simulink model "test1"  (R2015a)
settings: Solver=ode3  StartTime=0.0  StopTime=10.0  FixedStep=0.0001  RelTol=1e-3
settings Model: Creator=adelgayed60  LastModifiedBy=adelgayed60
settings OptimizationCC: InlineParams=on

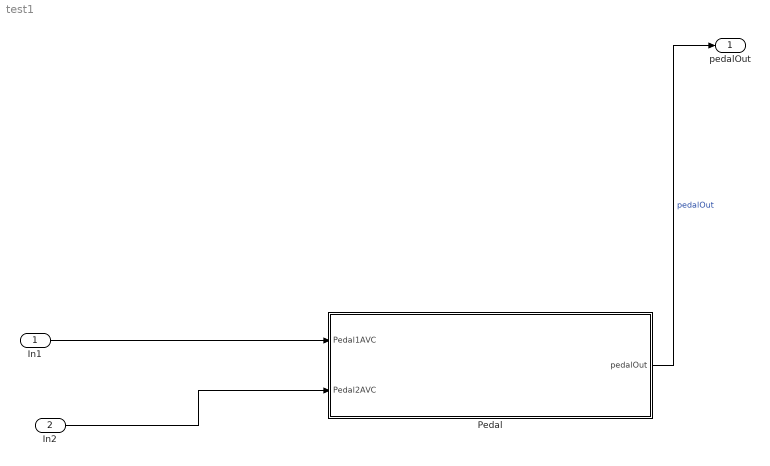
== system test1 ==
  In1 : Inport
  In2 : Inport  Port=2
  Pedal : Subsystem
  pedalOut : Outport
  wires:
  Pedal/1(pedalOut) -> pedalOut/1  "pedalOut"
  In1/1 -> Pedal/1(Pedal1AVC)
  In2/1 -> Pedal/2(Pedal2AVC)

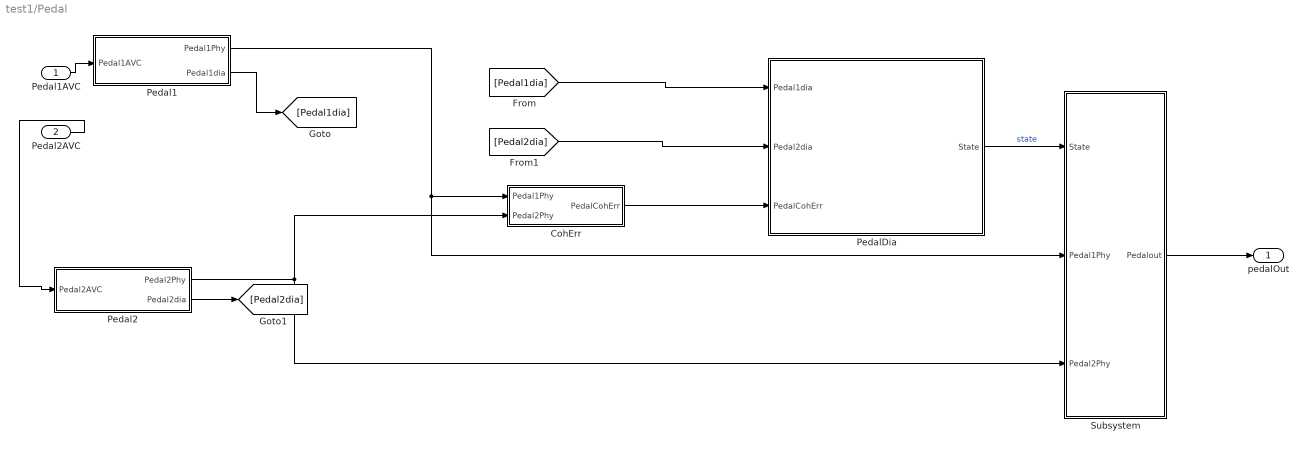
== system test1/Pedal ==
  Pedal1AVC : Inport
  Pedal2AVC : Inport  Port=2
  CohErr : Subsystem
  Pedal1 : Subsystem
  Pedal2 : Subsystem
  PedalDia : Subsystem
  Subsystem : Subsystem
  pedalOut : Outport
  wires:
  Pedal2/1(Pedal2Phy) -> CohErr/2(Pedal2Phy), Subsystem/3(Pedal2Phy)
  Subsystem/1(Pedalout) -> pedalOut/1
  Pedal2AVC/1 -> Pedal2/1(Pedal2AVC)
  Pedal2/2(Pedal2dia) -> [Pedal2dia]
  CohErr/1(PedalCohErr) -> PedalDia/3(PedalCohErr)
  [Pedal2dia] -> PedalDia/2(Pedal2dia)
  [Pedal1dia] -> PedalDia/1(Pedal1dia)
  PedalDia/1(State) -> Subsystem/1(State)  "state"
  Pedal1AVC/1 -> Pedal1/1(Pedal1AVC)
  Pedal1/2(Pedal1dia) -> [Pedal1dia]
  Pedal1/1(Pedal1Phy) -> Subsystem/2(Pedal1Phy), CohErr/1(Pedal1Phy)

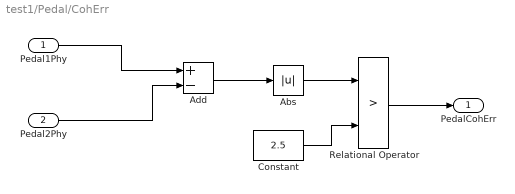
== system test1/Pedal/CohErr ==
  Pedal1Phy : Inport
  Pedal2Phy : Inport  Port=2
  Abs : Abs
  Add : Sum  Inputs=+-
  Constant : Constant  Value=2.5  OutDataTypeStr=single
  Relational Operator : RelationalOperator  Operator=>  OutDataTypeStr=boolean
  PedalCohErr : Outport
  wires:
  Pedal1Phy/1 -> Add/1
  Pedal2Phy/1 -> Add/2
  Add/1 -> Abs/1
  Abs/1 -> Relational Operator/1
  Relational Operator/1 -> PedalCohErr/1
  Constant/1 -> Relational Operator/2

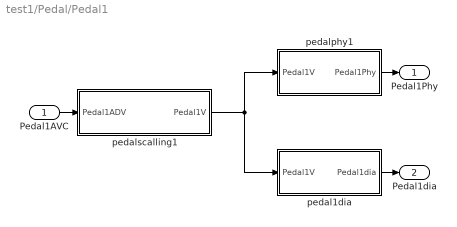
== system test1/Pedal/Pedal1 ==
  Pedal1AVC : Inport
  pedal1dia : Subsystem
  pedalphy1 : Subsystem
  pedalscalling1 : Subsystem
  Pedal1Phy : Outport
  Pedal1dia : Outport  Port=2
  wires:
  pedalscalling1/1(Pedal1V) -> pedal1dia/1(Pedal1V), pedalphy1/1(Pedal1V)
  pedal1dia/1(Pedal1dia) -> Pedal1dia/1
  pedalphy1/1(Pedal1Phy) -> Pedal1Phy/1
  Pedal1AVC/1 -> pedalscalling1/1(Pedal1ADV)

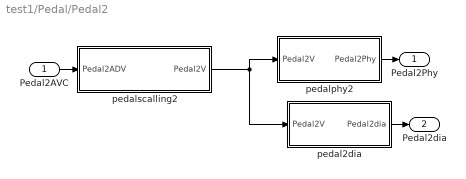
== system test1/Pedal/Pedal2 ==
  Pedal2AVC : Inport
  pedal2dia : Subsystem
  pedalphy2 : Subsystem
  pedalscalling2 : Subsystem
  Pedal2Phy : Outport
  Pedal2dia : Outport  Port=2
  wires:
  pedalscalling2/1(Pedal2V) -> pedal2dia/1(Pedal2V), pedalphy2/1(Pedal2V)
  pedalphy2/1(Pedal2Phy) -> Pedal2Phy/1
  pedal2dia/1(Pedal2dia) -> Pedal2dia/1
  Pedal2AVC/1 -> pedalscalling2/1(Pedal2ADV)

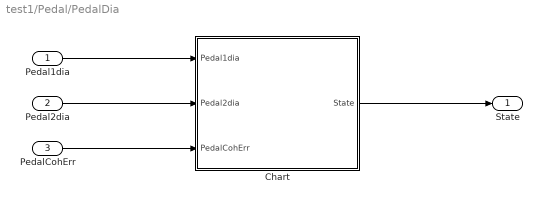
== system test1/Pedal/PedalDia ==
  Pedal1dia : Inport
  Pedal2dia : Inport  Port=2
  PedalCohErr : Inport  Port=3
  Chart : Stateflow chart  TreatAsAtomicUnit=on
  State : Outport
  wires:
  Pedal2dia/1 -> Chart/2(Pedal2dia)
  Pedal1dia/1 -> Chart/1(Pedal1dia)
  Chart/1(State) -> State/1
  PedalCohErr/1 -> Chart/3(PedalCohErr)

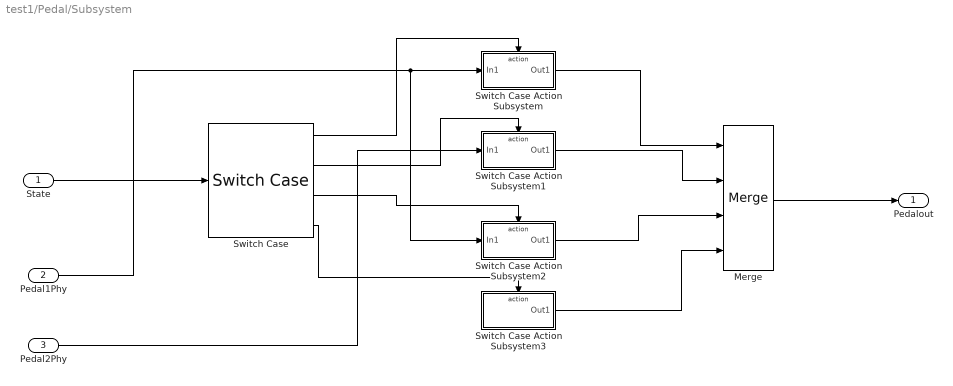
== system test1/Pedal/Subsystem ==
  State : Inport
  Pedal1Phy : Inport  Port=2
  Pedal2Phy : Inport  Port=3
  Merge : Merge  Inputs=4
  Switch Case : SwitchCase  CaseConditions={0,1,2,3}  ShowDefaultCase=off
  Switch Case Action Subsystem : Subsystem  TreatAsAtomicUnit=on
  Switch Case Action Subsystem1 : Subsystem  TreatAsAtomicUnit=on
  Switch Case Action Subsystem2 : Subsystem  TreatAsAtomicUnit=on
  Switch Case Action Subsystem3 : Subsystem  TreatAsAtomicUnit=on
  Pedalout : Outport
  wires:
  State/1 -> Switch Case/1
  Switch Case Action Subsystem/1(Out1) -> Merge/1
  Switch Case Action Subsystem1/1(Out1) -> Merge/2
  Switch Case Action Subsystem2/1(Out1) -> Merge/3
  Switch Case Action Subsystem3/1(Out1) -> Merge/4
  Switch Case/1 -> Switch Case Action Subsystem/Action
  Switch Case/2 -> Switch Case Action Subsystem1/Action
  Switch Case/3 -> Switch Case Action Subsystem2/Action
  Switch Case/4 -> Switch Case Action Subsystem3/Action
  Pedal1Phy/1 -> Switch Case Action Subsystem2/1(In1), Switch Case Action Subsystem/1(In1)
  Merge/1 -> Pedalout/1
  Pedal2Phy/1 -> Switch Case Action Subsystem1/1(In1)

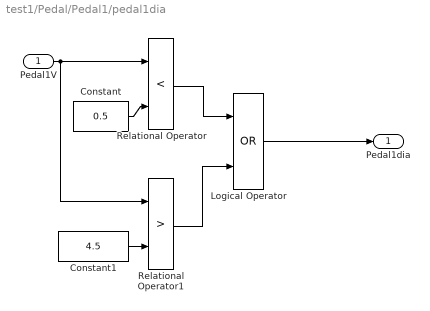
== system test1/Pedal/Pedal1/pedal1dia ==
  Pedal1V : Inport
  Constant : Constant  Value=0.5  OutDataTypeStr=single
  Constant1 : Constant  Value=4.5  OutDataTypeStr=single
  Logical Operator : Logic  Operator=OR  AllPortsSameDT=off  OutDataTypeStr=boolean
  Relational Operator : RelationalOperator  Operator=<  OutDataTypeStr=boolean
  Relational Operator1 : RelationalOperator  Operator=>  OutDataTypeStr=boolean
  Pedal1dia : Outport
  wires:
  Constant/1 -> Relational Operator/2
  Pedal1V/1 -> Relational Operator1/1, Relational Operator/1
  Constant1/1 -> Relational Operator1/2
  Logical Operator/1 -> Pedal1dia/1
  Relational Operator/1 -> Logical Operator/1
  Relational Operator1/1 -> Logical Operator/2

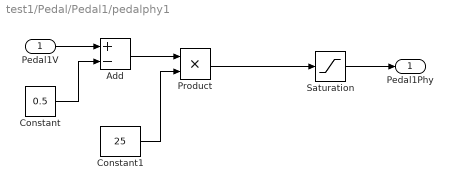
== system test1/Pedal/Pedal1/pedalphy1 ==
  Pedal1V : Inport
  Add : Sum  Inputs=+-
  Constant : Constant  Value=0.5  OutDataTypeStr=single
  Constant1 : Constant  Value=25  OutDataTypeStr=single
  Product : Product
  Saturation : Saturate  UpperLimit=100  LowerLimit=0  OutDataTypeStr=single
  Pedal1Phy : Outport
  wires:
  Pedal1V/1 -> Add/1
  Constant/1 -> Add/2
  Add/1 -> Product/1
  Constant1/1 -> Product/2
  Saturation/1 -> Pedal1Phy/1
  Product/1 -> Saturation/1

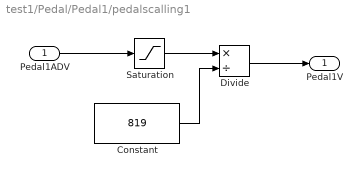
== system test1/Pedal/Pedal1/pedalscalling1 ==
  Pedal1ADV : Inport
  Constant : Constant  Value=819  OutDataTypeStr=uint16
  Divide : Product  Inputs=*/  OutDataTypeStr=single
  Saturation : Saturate  UpperLimit=4095  LowerLimit=0  OutDataTypeStr=uint16
  Pedal1V : Outport
  wires:
  Pedal1ADV/1 -> Saturation/1
  Saturation/1 -> Divide/1
  Constant/1 -> Divide/2
  Divide/1 -> Pedal1V/1

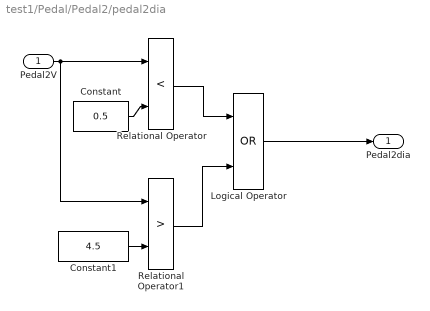
== system test1/Pedal/Pedal2/pedal2dia ==
  Pedal2V : Inport
  Constant : Constant  Value=0.5  OutDataTypeStr=single
  Constant1 : Constant  Value=4.5  OutDataTypeStr=single
  Logical Operator : Logic  Operator=OR  AllPortsSameDT=off  OutDataTypeStr=boolean
  Relational Operator : RelationalOperator  Operator=<  OutDataTypeStr=boolean
  Relational Operator1 : RelationalOperator  Operator=>  OutDataTypeStr=boolean
  Pedal2dia : Outport
  wires:
  Relational Operator1/1 -> Logical Operator/2
  Relational Operator/1 -> Logical Operator/1
  Logical Operator/1 -> Pedal2dia/1
  Constant1/1 -> Relational Operator1/2
  Pedal2V/1 -> Relational Operator/1, Relational Operator1/1
  Constant/1 -> Relational Operator/2

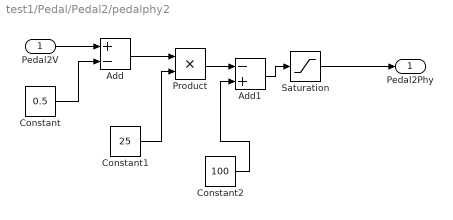
== system test1/Pedal/Pedal2/pedalphy2 ==
  Pedal2V : Inport
  Add : Sum  Inputs=+-
  Add1 : Sum  Inputs=-+
  Constant : Constant  Value=0.5  OutDataTypeStr=single
  Constant1 : Constant  Value=25  OutDataTypeStr=single
  Constant2 : Constant  Value=100  OutDataTypeStr=single
  Product : Product
  Saturation : Saturate  UpperLimit=100  LowerLimit=0  OutDataTypeStr=single
  Pedal2Phy : Outport
  wires:
  Constant1/1 -> Product/2
  Add/1 -> Product/1
  Constant/1 -> Add/2
  Pedal2V/1 -> Add/1
  Saturation/1 -> Pedal2Phy/1
  Product/1 -> Add1/1
  Constant2/1 -> Add1/2
  Add1/1 -> Saturation/1

== system test1/Pedal/Pedal2/pedalscalling2 ==
  Pedal2ADV : Inport
  Constant : Constant  Value=819  OutDataTypeStr=uint16
  Divide : Product  Inputs=*/  OutDataTypeStr=single
  Saturation : Saturate  UpperLimit=4095  LowerLimit=0  OutDataTypeStr=uint16
  Pedal2V : Outport
  wires:
  Divide/1 -> Pedal2V/1
  Constant/1 -> Divide/2
  Saturation/1 -> Divide/1
  Pedal2ADV/1 -> Saturation/1

== system test1/Pedal/Subsystem/Switch Case Action Subsystem ==
  In1 : Inport
  Action Port : ActionPort  ActionType=case
  Out1 : Outport
  wires:
  In1/1 -> Out1/1

== system test1/Pedal/Subsystem/Switch Case Action Subsystem1 ==
  In1 : Inport
  Action Port : ActionPort  ActionType=case
  Saturation : Saturate  UpperLimit=20  LowerLimit=0
  Out1 : Outport
  wires:
  In1/1 -> Saturation/1
  Saturation/1 -> Out1/1

== system test1/Pedal/Subsystem/Switch Case Action Subsystem2 ==
  In1 : Inport
  Action Port : ActionPort  ActionType=case
  Saturation : Saturate  UpperLimit=20  LowerLimit=0
  Out1 : Outport
  wires:
  In1/1 -> Saturation/1
  Saturation/1 -> Out1/1

== system test1/Pedal/Subsystem/Switch Case Action Subsystem3 ==
  Action Port : ActionPort  ActionType=case
  Constant : Constant  Value=0  OutDataTypeStr=single
  Out1 : Outport
  wires:
  Constant/1 -> Out1/1

== stateflow chart test1/Pedal/PedalDia/Chart ==
  state starting
    entry:
    State=uint8(0);
  state Pedal2
    entry:
    State=uint8(2);
  state Pedal1
    entry:
    State=uint8(1);
  state sturation
    entry:
    State=uint8(3);
  (default) -> starting
  (junction 1) -> starting [order 5]
  starting -> (junction 1)
  (junction 1) -> Pedal1 [order 2] : [Pedal1dia]
  (junction 1) -> Pedal2 [order 3] : [Pedal2dia]
  Pedal1 -> (junction 1)
  Pedal2 -> (junction 1)
  (junction 1) -> sturation [order 1] : [Pedal1dia&&Pedal2dia]
  (junction 1) -> sturation [order 4] : [PedalCohErr]
  sturation -> (junction 1)
  data: Pedal1dia input size=1; Pedal2dia input size=1; State output size=1; PedalCohErr input size=1
